simulink model "Block1112"  (R2016b)
settings: Solver=VariableStepAuto  StartTime=0.0  StopTime=10.0  RelTol=1e-3
libraries: simulink x6
settings Model: Creator=viett  LastModifiedBy=viett

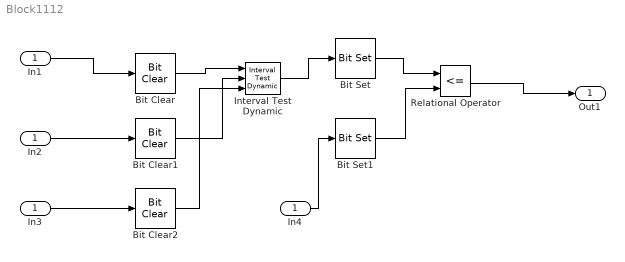
== system Block1112 ==
  In1 : Inport
  Bit Clear : simulink/Logic and Bit Operations/Bit Clear  iBit=0
  Bit Clear1 : simulink/Logic and Bit Operations/Bit Clear  iBit=0
  Bit Clear2 : simulink/Logic and Bit Operations/Bit Clear  iBit=0
  Bit Set : simulink/Logic and Bit Operations/Bit Set  iBit=0
  Bit Set1 : simulink/Logic and Bit Operations/Bit Set  iBit=0
  In2 : InportShadow
  In3 : InportShadow
  In4 : InportShadow
  Interval Test Dynamic : simulink/Logic and Bit Operations/Interval Test Dynamic  IntervalClosedRight=on  IntervalClosedLeft=on  OutDataTypeStr=boolean
  Relational Operator : RelationalOperator  Operator=<=  OutDataTypeStr=boolean  RndMeth=Simplest
  Out1 : Outport
  wires:
  Interval Test Dynamic/1 -> Bit Set/1
  Bit Set/1 -> Relational Operator/1
  Bit Clear/1 -> Interval Test Dynamic/1
  Bit Clear1/1 -> Interval Test Dynamic/2
  Bit Clear2/1 -> Interval Test Dynamic/3
  Bit Set1/1 -> Relational Operator/2
  Relational Operator/1 -> Out1/1
  In1/1 -> Bit Clear/1
  In2/1 -> Bit Clear1/1
  In3/1 -> Bit Clear2/1
  In4/1 -> Bit Set1/1
